simulink model "FollowTrajectory"  (R2023b)
settings: Solver=VariableStepAuto  StartTime=0.0  StopTime=50.0  RelTol=1e-3
model workspace (MAT data in the model file):
  t = Simulink.Parameter
  t.DataType = 'auto'
  t.Complexity = 'real'
  t.Dimensions = [0 0]
settings Model: Creator=haluk  LastModifiedBy=Baki
settings DebuggingCC: UnconnectedInputMsg=warning  UnconnectedOutputMsg=warning  UnconnectedLineMsg=warning
settings ModelReferenceCC: EnableRefExpFcnMdlSchedulingChecks=on
settings RTWCC: DLArmComputeVersion=19.05

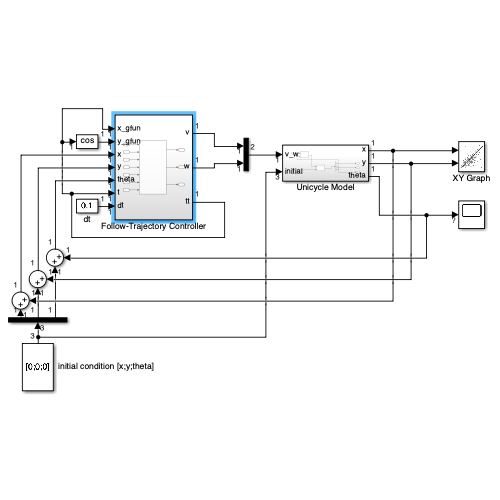
[thumbnail: Simulink's stored preview of the top-level diagram]
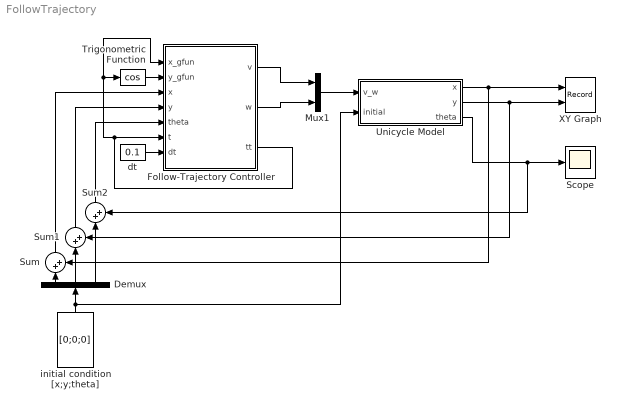
== system FollowTrajectory ==
  Demux : Demux  Outputs=3
  Follow-Trajectory Controller : Subsystem
  Mux1 : Mux  Inputs=2
  Scope : Scope
  Sum : Sum  Inputs=|++
  Sum1 : Sum  Inputs=|++
  Sum2 : Sum  Inputs=|++
  Trigonometric Function : Trigonometry  Operator=cos
  Unicycle Model : Subsystem
  XY Graph : Record  FileSettingsInternal="{\"entries\":[{\"content\":{\"excelSettings\":{\"content\":{},\"type\":\"Streamout.ExcelSettings\"}},\"type\":\"Streamout.FileSettingStorage\",\"uuid\":\"\"}],\"packageUris\":[\"http:\\/\\/schema.mathworks.com\\/mf0\\/streamout_blocks\\/R2020a\"],\"version\":\"1.0\"}"  Layout=[1 1]  SignalsInternal="{\"entries\":[{\"content\":{\"signals\":[{\"content\":{\"blockPath\":[],\"dimensions\":[1],\"domain\":\"\",\"lineColor\":\"#a2142f\",\"plots\":[1],\"port\":1,\"signalID\":8,\"signalName\":\"XY Graph:1\"},\"type\":\"RecordBlkView.Signal\",\"uuid\":\"\"},{\"content\":{\"blockPath\":[],\"dimensions\":[1],\"domain\":\"\",\"lineColor\":\"#139fff\",\"plots\":[1],\"port\":2,\"signalID\":11,\"signalName\":\"XY Graph:2\"},\"type\":\"RecordBlkView.Signal\",\"uuid\":\"\"}]},\"type\":\"RecordBlkView.InputSignals\",\"uuid\":\"\"}],\"packageUris\":[\"http:\\/\\/schema.mathworks.com\\/mf0\\/streamout_blocks\\/R2020a\"],\"version\":\"1.0\"}"  VisualizationBindings="{\"xyplotplugin\":{\"info\":[{\"series\":[{\"bindingParametersList\":[{\"parameter\":\"X-Axis\",\"signalID\":8,\"signalName\":\"XY Graph:1\"},{\"parameter\":\"Y-Axis\",\"signalID\":11,\"signalName\":\"XY Graph:2\"}],\"seriesID\":38499}],\"subplotID\":1}]}}"  CompatibilityTag=XY  st=-1
  dt : Constant  Value=0.1
  initial condition [x;y;theta] : Constant  Value=[0;0;0]
  wires:
  Unicycle Model/1(x) -> Sum/2, XY Graph/1
  Unicycle Model/2(y) -> Sum1/2, XY Graph/2
  Unicycle Model/3(theta) -> Sum2/2, Scope/1
  Mux1/1 -> Unicycle Model/1(v_w)
  Follow-Trajectory Controller/1(v) -> Mux1/1
  Follow-Trajectory Controller/2(w) -> Mux1/2
  Trigonometric Function/1 -> Follow-Trajectory Controller/2(y_gfun)
  dt/1 -> Follow-Trajectory Controller/7(dt)
  Follow-Trajectory Controller/3(tt) -> Follow-Trajectory Controller/6(t), Follow-Trajectory Controller/1(x_gfun), Trigonometric Function/1
  initial condition [x;y;theta]/1 -> Unicycle Model/2(initial), Demux/1
  Demux/1 -> Sum/1
  Sum2/1 -> Follow-Trajectory Controller/5(theta)
  Sum1/1 -> Follow-Trajectory Controller/4(y)
  Sum/1 -> Follow-Trajectory Controller/3(x)
  Demux/3 -> Sum2/1
  Demux/2 -> Sum1/1

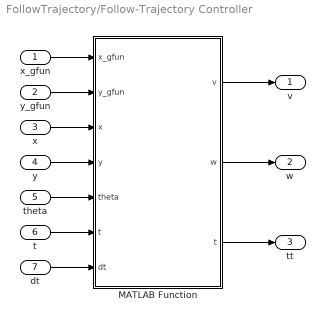
== system FollowTrajectory/Follow-Trajectory Controller ==
  x_gfun : Inport
  y_gfun : Inport  Port=2
  x : Inport  Port=3
  y : Inport  Port=4
  theta : Inport  Port=5
  t : Inport  Port=6
  dt : Inport  Port=7
  MATLAB Function : MATLAB Function  TreatAsAtomicUnit=on
  v : Outport
  w : Outport  Port=2
  tt : Outport  Port=3
  wires:
  MATLAB Function/1(v) -> v/1
  MATLAB Function/2(w) -> w/1
  x_gfun/1 -> MATLAB Function/1(x_gfun)
  y_gfun/1 -> MATLAB Function/2(y_gfun)
  x/1 -> MATLAB Function/3(x)
  y/1 -> MATLAB Function/4(y)
  theta/1 -> MATLAB Function/5(theta)
  t/1 -> MATLAB Function/6("t ")
  dt/1 -> MATLAB Function/7(dt)
  MATLAB Function/3(t) -> tt/1

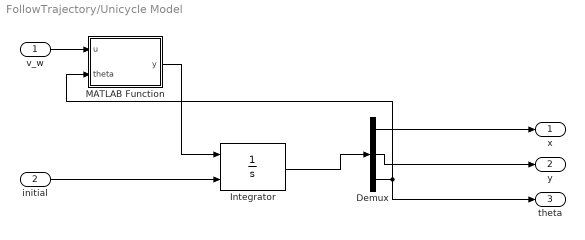
== system FollowTrajectory/Unicycle Model ==
  v_w : Inport
  initial : Inport  Port=2
  Demux : Demux  Outputs=3
  Integrator : Integrator  InitialConditionSource=external
  MATLAB Function : MATLAB Function  TreatAsAtomicUnit=on
  x : Outport
  y : Outport  Port=2
  theta : Outport  Port=3
  wires:
  MATLAB Function/1(y) -> Integrator/1
  Demux/3 -> theta/1, MATLAB Function/2(theta)
  Integrator/1 -> Demux/1
  Demux/1 -> x/1
  initial/1 -> Integrator/2
  v_w/1 -> MATLAB Function/1(u)
  Demux/2 -> y/1

== matlab function FollowTrajectory/Unicycle Model/MATLAB Function ==
  data: u input; y output; theta input
function y = fcn(u, theta)


v = u(1);
w = u(2);

y = [v*cos(theta); v*sin(theta); w];

== matlab function FollowTrajectory/Follow-Trajectory Controller/MATLAB Function ==
  data: x_gfun input; y_gfun input; x input; y input; v output; theta input; w output; t input; dt input; t output
function [v,w,t]= fcn(x_gfun, y_gfun, x, y, theta,t ,dt)

Kv = 1.0;
Ki = 1.0;
Kh = 1.0;

t = t + dt;

x_g = x_gfun;
y_g = y_gfun;

% Hız ve dönüş açısı hesaplama
e = sqrt((x_g - x)^2 + (y_g - y)^2) - d;
vt = Kv * e + Ki * (e*t - e*(t-dt)); %integral(e,t-dt,t);
theta_g = atan2(y_g - y, x_g - x);
wt = Kh * (atan2(sin(theta_g - theta), cos(theta_g - theta)));

v = vt;
w = wt;
